simulink model "trial"  (R2020b)
settings: Solver=VariableStepAuto  StartTime=0.0  StopTime=10.0  RelTol=1e-3
model workspace (MAT data in the model file):
  L = 1
  g = 9.81
settings Model: Creator=divyaprakash  LastModifiedBy=divyaprakash

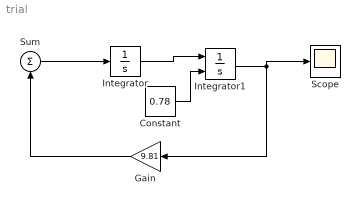
== system trial ==
  Constant : Constant  Value=0.78
  Gain : Gain  Gain=9.81
  Integrator : Integrator
  Integrator1 : Integrator  InitialConditionSource=external  InitialCondition=0.7854
  Scope : Scope
  Sum : Sum  Inputs=|+
  wires:
  Sum/1 -> Integrator/1
  Integrator/1 -> Integrator1/1
  Integrator1/1 -> Scope/1, Gain/1
  Gain/1 -> Sum/1
  Constant/1 -> Integrator1/2
